simulink model "Pancake_FTC_Mine"  (Simulink 7.6)
settings: Solver=ode45  StartTime=0.0  StopTime=6000  MaxStep=0.1  RelTol=1e-5
InitFcn:
  | initMine;
StopFcn:
  | save('mySimResult.mat');
  | %plot_sim_result
values from neighbouring files (symbols this model uses):
  A = [0 0 0 0 0 0 0 0 0 0 0 0 ... (576 elements, 24x24)]    [sys3.mat]
  Aw = [-0.00835261575623 0 0 0 0 0 0 0 0 0 0 0 ... (339889 elements, 583x583)]    [W_filt.mat]
  B = [0 0 0 0 0 0 0 0 0 0 0 0 ... (120 elements, 24x5)]    [sys3.mat]
  Bw = [0 0 0 0 0 0 0 0 0 0 0 0 ... (2915 elements, 583x5)]    [W_filt.mat]
  C = [0.000235530581915 0.000235530581915 0.000235530581915 0.000235530581915 0.000235530581915 0.000425739149389 -0.000425739149389 0 -0.000425739149389 0.000425739149389 0.000425739149389 0.000425739149389 ... (120 elements, 5x24)]    [sys3.mat]
  Cw = [-0.0221066892306 0 0 0 0 5.33760623616e-06 0 0 0 0 -0.0228699604243 0 ... (2915 elements, 5x583)]    [W_filt.mat]    (also in initMine.m = 1e4*Cw; init_fd.m = 1e4*Cw)
  Dw = [0 0.337392530431 132.837452972 1.686188572 -0.0653172616444 0.337391892996 0 -132.837304132 -0.169967704957 0.647988894412 1 1 ... (25 elements, 5x5)]    [W_filt.mat]    (also in initMine.m = 1e4*Dw; init_fd.m = 1e4*Dw)
  H = [6.82787147858 26.1817309148 305.949237812 11.1181420095 7.63670516742 468.011692264 -23.0078717509 10.568259224 -36.8457797424 149946.441442 46.1828079041 -6736.97140431 ... (120 elements, 24x5)]    [W_filt.mat]
  m = length(Y_mat)/3    [PID_PD_4.m]    (also in Sam_FD.m = block.InputPort(2).Dimensions; myFD.m = block.OutputPort(1).Dimensions; myFD2.m = block.OutputPort(1).Dimensions; sys3.mat = 5)
  n = n/2    [initMine.m]    (also in init_fd.m; sys3.mat = 12)
  w = zeros(q,1)    [init.m]    (also in initMine.m; init_fd.m; plant_model.m = inp(2*n+m+1:2*n+m+q); plant_output.m = inp(2*n+m+1:2*n+m+q))
  x0 = zeros(2*n,1)    [init.m]    (also in initMine.m; init_fd.m = randn(2*n,1))
  yref = [1; 2; 0.5; -2; -3]    [init.m]    (also in initMine.m)
settings Model: Creator=Yao Hong Kok  LastModifiedBy=SCG
settings DebuggingCC: StrictBusMsg=Warning
settings ModelReferenceCC: UpdateModelReferenceTargets=IfOutOfDate
settings SFSimCC: SFSimEcho=off  SimParseCustomCode=off

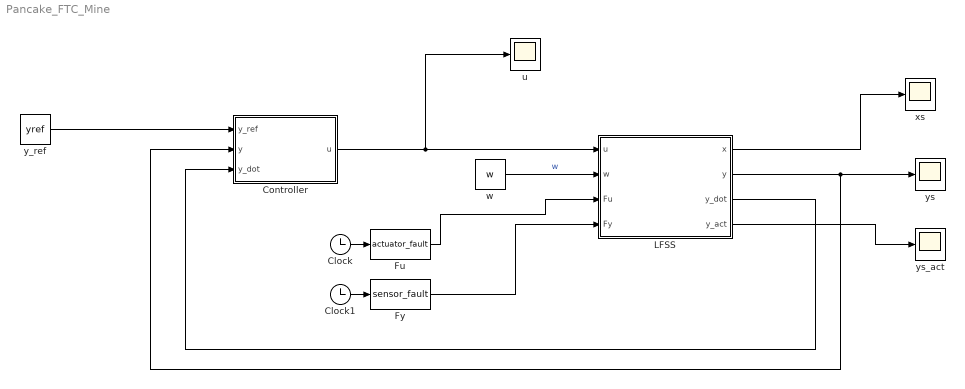
== system Pancake_FTC_Mine ==
  Clock : Clock
      settings: Decimation=10
  Clock1 : Clock
      settings: Decimation=10
  Controller : Subsystem
  Fu : MATLABFcn  MATLABFcn=actuator_fault
  Fy : MATLABFcn  MATLABFcn=sensor_fault
  LFSS : Subsystem
  u : Scope
      settings: SaveName=us
  w : Constant  Value=w
  xs : Scope
      settings: SaveName=xs
  y_ref : Constant  Value=yref
  ys : Scope
      settings: YMin=-140  YMax=10  SaveName=ys
  ys_act : Scope
      settings: YMax=27.5  SaveName=ys4
  wires:
  LFSS/1(x) -> xs/1
  LFSS/2(y) -> ys/1, Controller/2(y)
  w/1 -> LFSS/2(w)  "w"
  Clock/1 -> Fu/1
  Fu/1 -> LFSS/3(Fu)
  Clock1/1 -> Fy/1
  Fy/1 -> LFSS/4(Fy)
  Controller/1(u) -> LFSS/1(u), u/1
  y_ref/1 -> Controller/1(y_ref)
  LFSS/3(y_dot) -> Controller/3(y_dot)
  LFSS/4(y_act) -> ys_act/1

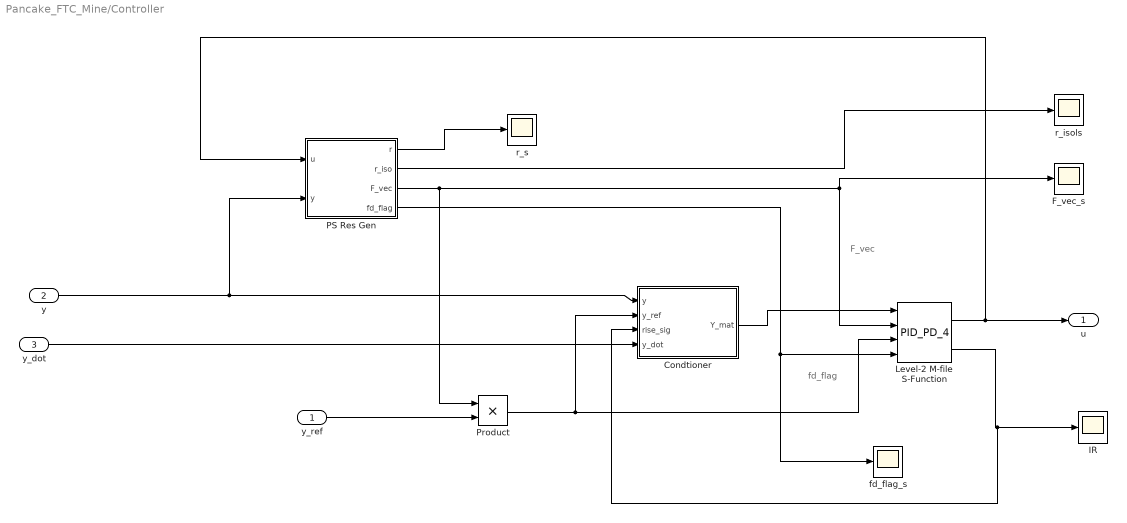
== system Pancake_FTC_Mine/Controller ==
  note: F_vec
  note: fd_flag
  y_ref : Inport
  y : Inport  Port=2
  y_dot : Inport  Port=3
  Condtioner : Subsystem
  F_vec_s : Scope
      settings: SaveName=F_vec_s
  IR : Scope
      settings: TimeRange=40  YMin=0  YMax=1  SaveName=IR_s
  Level-2 M-file S-Function : M-S-Function  FunctionName=PID_PD_4
  PS Res Gen : Subsystem
  Product : Product  RndMeth=Zero
  fd_flag_s : Scope
      settings: SaveName=fd_flag_s
  r_isols : Scope
      settings: SaveName=r_isol_s
  r_s : Scope
      settings: YMin=-0.00045  YMax=0.00025  SaveName=rl_s
  u : Outport
  wires:
  Condtioner/1(Y_mat) -> Level-2 M-file S-Function/1
  Level-2 M-file S-Function/1 -> u/1, PS Res Gen/1(u)
  y/1 -> Condtioner/1(y), PS Res Gen/2(y)
  y_dot/1 -> Condtioner/4(y_dot)
  PS Res Gen/4(fd_flag) -> Level-2 M-file S-Function/4, fd_flag_s/1
  PS Res Gen/3(F_vec) -> Level-2 M-file S-Function/2, F_vec_s/1, Product/1
  PS Res Gen/2(r_iso) -> r_isols/1
  y_ref/1 -> Product/2
  Product/1 -> Level-2 M-file S-Function/3, Condtioner/2(y_ref)
  PS Res Gen/1(r) -> r_s/1
  Level-2 M-file S-Function/2 -> Condtioner/3(rise_sig), IR/1

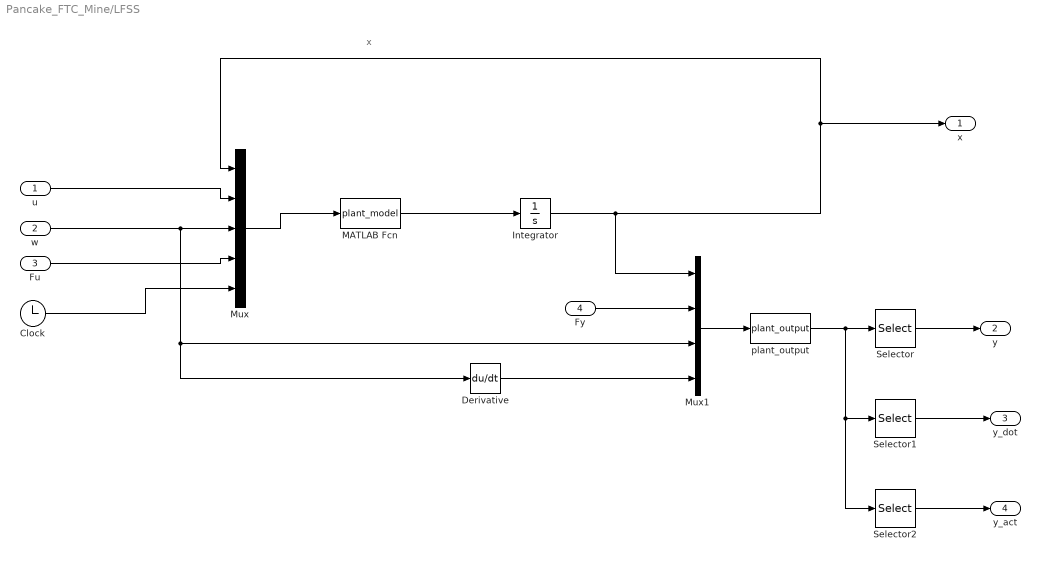
== system Pancake_FTC_Mine/LFSS ==
  note: x
  u : Inport
  w : Inport  Port=2
  Fu : Inport  Port=3
  Fy : Inport  Port=4
  Clock : Clock
  Derivative : Derivative
  Integrator : Integrator  InitialCondition=x0
  MATLAB Fcn : MATLABFcn  MATLABFcn=plant_model  OutputDimensions=24
  Mux : Mux  Inputs=5
  Mux1 : Mux
  Selector : Selector  InputPortWidth=3*m  IndexOptions=Index vector (dialog)  Indices=[1:m]  OutputSizes=1
  Selector1 : Selector  InputPortWidth=3*m  IndexOptions=Index vector (dialog)  Indices=[m+1:2*m]  OutputSizes=1
  Selector2 : Selector  InputPortWidth=3*m  IndexOptions=Index vector (dialog)  Indices=[2*m+1:3*m]  OutputSizes=1
  plant_output : MATLABFcn  MATLABFcn=plant_output
  x : Outport
  y : Outport  Port=2
  y_dot : Outport  Port=3
  y_act : Outport  Port=4
  wires:
  MATLAB Fcn/1 -> Integrator/1
  Mux/1 -> MATLAB Fcn/1
  Integrator/1 -> Mux/1, x/1, Mux1/1
  u/1 -> Mux/2
  w/1 -> Mux/3, Mux1/3, Derivative/1
  Fu/1 -> Mux/4
  Mux1/1 -> plant_output/1
  Fy/1 -> Mux1/2
  Clock/1 -> Mux/5
  Derivative/1 -> Mux1/4
  plant_output/1 -> Selector/1, Selector1/1, Selector2/1
  Selector/1 -> y/1
  Selector1/1 -> y_dot/1
  Selector2/1 -> y_act/1

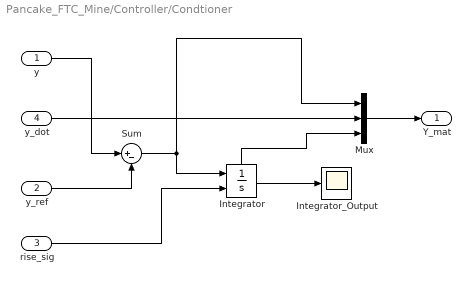
== system Pancake_FTC_Mine/Controller/Condtioner ==
  y : Inport
  y_ref : Inport  Port=2
  rise_sig : Inport  Port=3
  y_dot : Inport  Port=4
  Integrator : Integrator  ExternalReset=either  ShowStatePort=on
  Integrator_Output : Scope
      settings: SaveName=ys2
  Mux : Mux  Inputs=3
  Sum : Sum  Inputs=|+-
  Y_mat : Outport
  wires:
  Mux/1 -> Y_mat/1
  y/1 -> Sum/1
  y_ref/1 -> Sum/2
  Sum/1 -> Integrator/1, Mux/1
  rise_sig/1 -> Integrator/2
  Integrator/State -> Mux/3
  Integrator/1 -> Integrator_Output/1
  y_dot/1 -> Mux/2

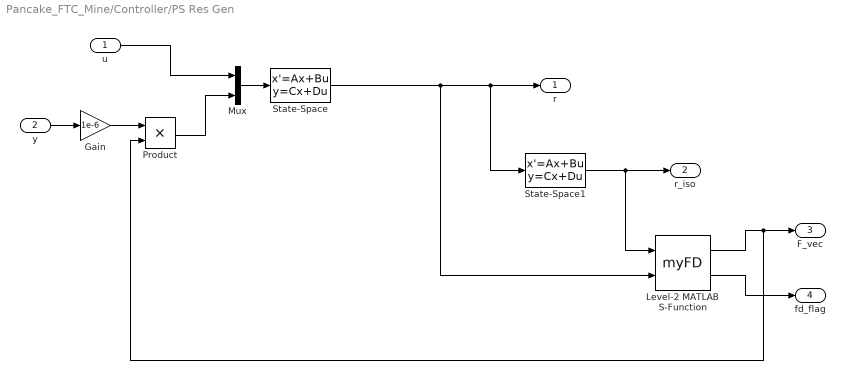
== system Pancake_FTC_Mine/Controller/PS Res Gen ==
  u : Inport
  y : Inport  Port=2
  Gain : Gain  Gain=1e-6
  Level-2 MATLAB S-Function : M-S-Function  FunctionName=myFD
  Mux : Mux  Inputs=2
  Product : Product  RndMeth=Zero
  State-Space : StateSpace  A=A-H*C  B=[B H]  C=C  D=[zeros(m) eye(m)]  X0=zeros(2*n,1)
  State-Space1 : StateSpace  A=Aw  B=Bw  C=Cw  D=Dw  X0=zeros(length(Aw),1)
  r : Outport
  r_iso : Outport  Port=2
  F_vec : Outport  Port=3
  fd_flag : Outport  Port=4
  wires:
  Mux/1 -> State-Space/1
  u/1 -> Mux/1
  State-Space/1 -> r/1, State-Space1/1, Level-2 MATLAB S-Function/2
  State-Space1/1 -> r_iso/1, Level-2 MATLAB S-Function/1
  Level-2 MATLAB S-Function/2 -> fd_flag/1
  Product/1 -> Mux/2
  Level-2 MATLAB S-Function/1 -> F_vec/1, Product/2
  Gain/1 -> Product/1
  y/1 -> Gain/1
